simulink model "Restore_changes"  (R2022b)
settings: Solver=VariableStepAuto  StartTime=0.0  StopTime=10.0  RelTol=1e-3
undefined symbols (not defined in the file): Amplifier, DiscIntNeverNeededParam, K_d_yawrate, K_dsteering, k_speed, k_stanley
libraries: CarMaker4SL x19, simulink x7
settings Model: Creator=Admin  LastModifiedBy=Admin

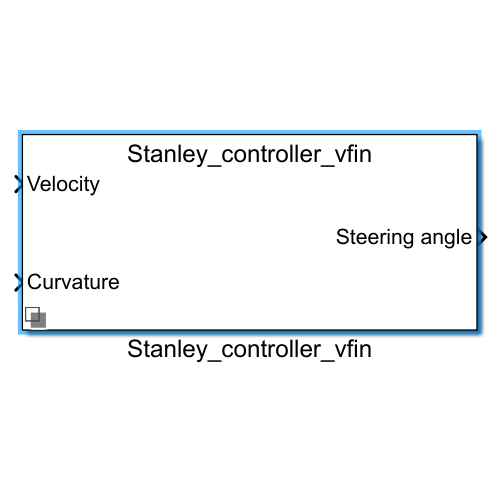
[thumbnail: Simulink's stored preview of the top-level diagram]
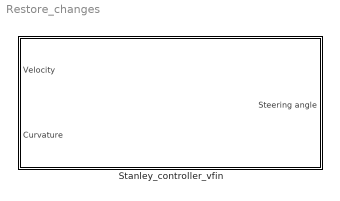
== system Restore_changes ==
  Stanley_controller_vfin : Subsystem  Variant=on  VariantControlMode=label  VariantControl=Choice  LabelModeActiveChoice=Choice

== system Restore_changes/Stanley_controller_vfin ==
  Velocity : Inport
  Curvature : Inport  Port=2
  Stanley_controller_vfin : Subsystem  Variant=on  VariantControlMode=label  VariantControl=Choice  LabelModeActiveChoice=Choice
  Steering angle : Outport

== system Restore_changes/Stanley_controller_vfin/Stanley_controller_vfin ==
  Velocity : Inport
  Curvature : Inport  Port=2
  Stanley_standfort controller : Subsystem  VariantControl=Choice
  Steering angle : Outport

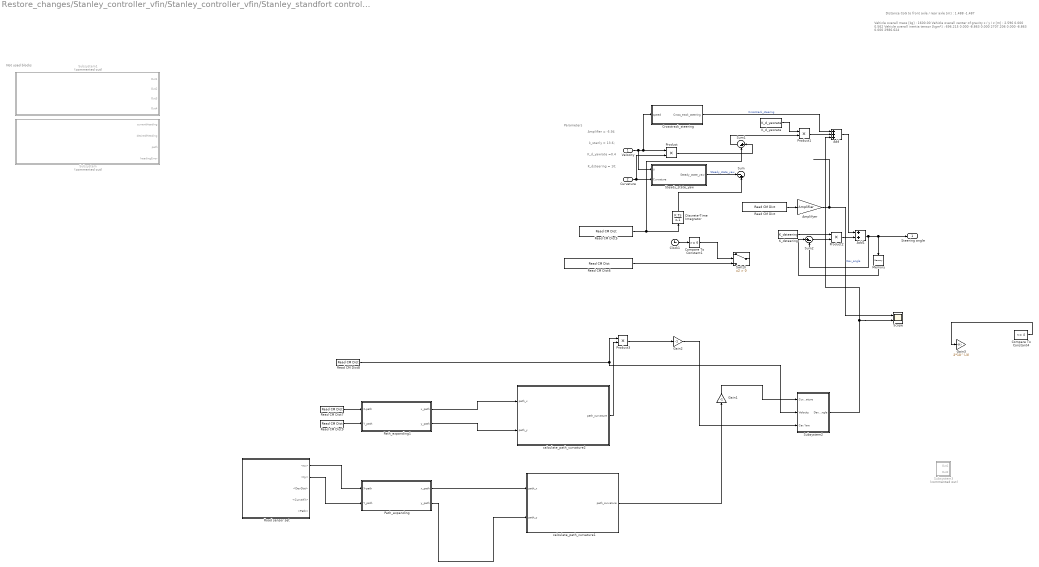
== system Restore_changes/Stanley_controller_vfin/Stanley_controller_vfin/Stanley_standfort controller ==
  note: Parameters
  note: K_dsteering = 10;
  note: Amplifier = -5.94
  note: K_d_yawrate =0.4
  note: Vehicle overall mass [kg] 	: 	1600.00
      |
      |  Vehicle overall center of gravity x / y / z [m] 	: 	2.596	0.000	0.562
      |
      |  Vehicle overall inertia tensor [kgm²] 	: 	696.215	0.000	-8.863
      |  	 									0.000	2707.206	0.000
      |  	 									-8.863	0.000	2986.624
  note: Distance CoG to front axle / rear axle [m] : 1.488 -1.487
  note: k_stanly = 13.6;
  note: Not used blocks
  Velocity : Inport
  Curvature : Inport  Port=2
  " Path_expanding" : Subsystem
  " Path_expanding1" : Subsystem
  Add : Sum  Inputs=+++
  Add1 : Sum
  Amplifyer : Gain  Gain=Amplifier
  Clock1 : Clock
  Compare To Constant1 : simulink/Logic and Bit Operations/Compare To Constant  relop=>=  const=6  OutDataTypeStr=boolean
  Compare To Constant4 : simulink/Logic and Bit Operations/Compare To Constant  relop=<=  const=4  OutDataTypeStr=boolean
  Crosstrack_steering : Subsystem
  Discrete-Time Integrator : DiscreteIntegrator  SampleTime=-1  ICPrevOutput=DiscIntNeverNeededParam  ICPrevScaledInput=DiscIntNeverNeededParam
  Gain1 : Gain  Gain=-1
  Gain2 : Gain  Gain=-1
  Gain3 : Gain  Gain=2*10^(-3)
  K_d_yawrate : Constant  Value=K_d_yawrate
  K_dsteering : Constant  Value=K_dsteering
  Memory : Memory  LinearizeAsDelay=on
  Product{,1..3} (4 alike) : Product
  Read CM Dict : CarMaker4SL/Read CM Dict  xname=Sensor.Road.VehSensor_0.Path.DevAng  xsync=off  xstime=Continuous
  Read CM Dict5 : CarMaker4SL/Read CM Dict  xname=Car.YawRate  xsync=off  xstime=Continuous
  Read CM Dict6 : CarMaker4SL/Read CM Dict  xname=Sensor.Road.VehSensor_0.Path.CurveXY  xsync=off  xstime=Continuous
  Read CM Dict7 : CarMaker4SL/Read CM Dict  xname=Car.Gen.tx  xsync=off  xstime=Continuous
  Read CM Dict8 : CarMaker4SL/Read CM Dict  xname=Vhcl.v  xsync=off  xstime=Continuous
  Read CM Dict9 : CarMaker4SL/Read CM Dict  xname=Car.Gen.ty  xsync=off  xstime=Continuous
  Road sensor set : Subsystem  Variant=on  VariantControlMode=label  VariantControl=Choice  LabelModeActiveChoice=Choice
  Scope : Scope  NumInputPorts=2
  Steady_state_yaw : Subsystem
  Subsystem : Subsystem  Commented=on
  Subsystem1 : Subsystem  Commented=on
  Subsystem2 : Subsystem
  Subsystem3 : Subsystem  Commented=on
  Sum : Sum  Inputs=|-+
  Sum1 : Sum  Inputs=|+-
  Sum2 : Sum  Inputs=|+-
  Switch : Switch  Criteria=u2 > Threshold  SaturateOnIntegerOverflow=off  InputSameDT=off
  calculate_path_curvature1 : MATLAB Function  TreatAsAtomicUnit=on  VariantControl=Choice
  calculate_path_curvature2 : MATLAB Function  TreatAsAtomicUnit=on  VariantControl=Choice
  Steering angle : Outport
  wires:
  Read CM Dict5/1 -> Discrete-Time Integrator/1, Sum1/2
  Velocity/1 -> Crosstrack_steering/1(speed), Product/1, Steady_state_yaw/1(V)
  Curvature/1 -> Steady_state_yaw/2(Curvature), Product/2
  Crosstrack_steering/1(Cross_track_steering) -> Add/1  "Crosstrack_steering"
  Product/1 -> Sum1/1
  Steady_state_yaw/1(Steady_state_yaw) -> Sum/1  "Steady_state_yaw"
  Discrete-Time Integrator/1 -> Sum/2
  Sum1/1 -> Product1/2
  K_d_yawrate/1 -> Product1/1
  Product1/1 -> Add/2
  Read CM Dict/1 -> Amplifyer/1
  Amplifyer/1 -> Scope/1  "Dev_angle"
  K_dsteering/1 -> Product2/1
  Sum2/1 -> Product2/2
  Add/1 -> Add1/1
  Product2/1 -> Add1/2
  Add1/1 -> Memory/1, Steering angle/1, Sum2/2
  Memory/1 -> Sum2/1
  Read CM Dict6/1 -> Switch/3
  Read CM Dict8/1 -> Product3/1, Subsystem2/2(Velocity)
  Road sensor set/1(<tx>) -> " Path_expanding"/1(X-path)
  Road sensor set/2(<ty>) -> " Path_expanding"/2(Y_path)
  " Path_expanding"/1(x_path) -> calculate_path_curvature1/1(path_x)
  " Path_expanding"/2(y_path) -> calculate_path_curvature1/2(path_y)
  calculate_path_curvature1/1(path_curvature) -> Gain1/1
  Subsystem2/1(Dev_angle) -> Add/3, Scope/2
  Clock1/1 -> Compare To Constant1/1
  Compare To Constant1/1 -> Switch/2
  Compare To Constant4/1 -> Gain3/1
  Gain1/1 -> Subsystem2/1(Curvature)
  " Path_expanding1"/1(x_path) -> calculate_path_curvature2/1(path_x)
  " Path_expanding1"/2(y_path) -> calculate_path_curvature2/2(path_y)
  Read CM Dict7/1 -> " Path_expanding1"/1(X-path)
  Read CM Dict9/1 -> " Path_expanding1"/2(Y_path)
  calculate_path_curvature2/1(path_curvature) -> Product3/2
  Product3/1 -> Gain2/1
  Gain2/1 -> Subsystem2/3(Car.Yaw)

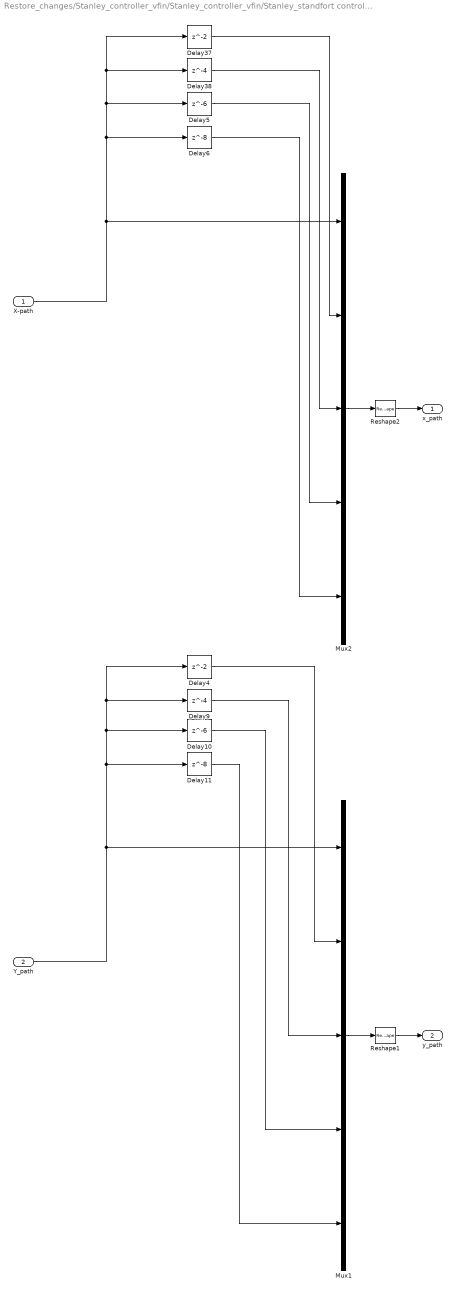
== system Restore_changes/Stanley_controller_vfin/Stanley_controller_vfin/Stanley_standfort controller/ Path_expanding ==
  X-path : Inport
  Y_path : Inport  Port=2
  Delay10 : Delay  DelayLength=6
  Delay11 : Delay  DelayLength=8
  Delay37 : Delay
  Delay38 : Delay  DelayLength=4
  Delay4 : Delay
  Delay5 : Delay  DelayLength=6
  Delay6 : Delay  DelayLength=8
  Delay9 : Delay  DelayLength=4
  Mux1 : Mux  Inputs=5
  Mux2 : Mux  Inputs=5
  Reshape1 : Reshape  OutputDimensionality=Customize  OutputDimensions=[1,5]
  Reshape2 : Reshape  OutputDimensionality=Customize  OutputDimensions=[1,5]
  x_path : Outport
  y_path : Outport  Port=2
  wires:
  X-path/1 -> Mux2/1, Delay38/1, Delay37/1, Delay5/1, Delay6/1
  Y_path/1 -> Mux1/1, Delay4/1, Delay9/1, Delay10/1, Delay11/1
  Delay5/1 -> Mux2/4
  Delay37/1 -> Mux2/2
  Delay6/1 -> Mux2/5
  Delay38/1 -> Mux2/3
  Mux1/1 -> Reshape1/1
  Reshape1/1 -> y_path/1
  Delay4/1 -> Mux1/2
  Delay9/1 -> Mux1/3
  Delay10/1 -> Mux1/4
  Delay11/1 -> Mux1/5
  Reshape2/1 -> x_path/1
  Mux2/1 -> Reshape2/1

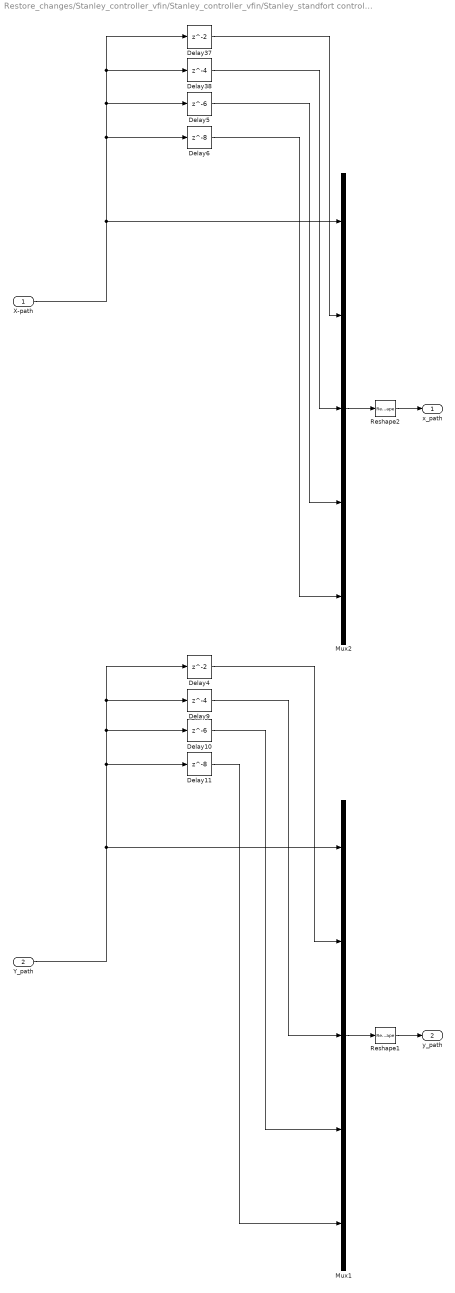
== system Restore_changes/Stanley_controller_vfin/Stanley_controller_vfin/Stanley_standfort controller/ Path_expanding1 ==
  X-path : Inport
  Y_path : Inport  Port=2
  Delay10 : Delay  DelayLength=6
  Delay11 : Delay  DelayLength=8
  Delay37 : Delay
  Delay38 : Delay  DelayLength=4
  Delay4 : Delay
  Delay5 : Delay  DelayLength=6
  Delay6 : Delay  DelayLength=8
  Delay9 : Delay  DelayLength=4
  Mux1 : Mux  Inputs=5
  Mux2 : Mux  Inputs=5
  Reshape1 : Reshape  OutputDimensionality=Customize  OutputDimensions=[1,5]
  Reshape2 : Reshape  OutputDimensionality=Customize  OutputDimensions=[1,5]
  x_path : Outport
  y_path : Outport  Port=2
  wires:
  Mux2/1 -> Reshape2/1
  Reshape2/1 -> x_path/1
  Delay11/1 -> Mux1/5
  Delay10/1 -> Mux1/4
  Delay9/1 -> Mux1/3
  Delay4/1 -> Mux1/2
  Reshape1/1 -> y_path/1
  Mux1/1 -> Reshape1/1
  Delay38/1 -> Mux2/3
  Delay6/1 -> Mux2/5
  Delay37/1 -> Mux2/2
  Delay5/1 -> Mux2/4
  Y_path/1 -> Delay11/1, Delay10/1, Delay9/1, Delay4/1, Mux1/1
  X-path/1 -> Delay6/1, Delay5/1, Delay37/1, Delay38/1, Mux2/1

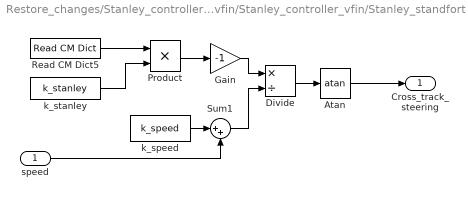
== system Restore_changes/Stanley_controller_vfin/Stanley_controller_vfin/Stanley_standfort controller/Crosstrack_steering ==
  speed : Inport
  Atan : Trigonometry  Operator=atan
  Divide : Product  Inputs=*/
  Gain : Gain  Gain=-1
  Product : Product
  Read CM Dict5 : CarMaker4SL/Read CM Dict  xname=Car.Road.Path.DevDist  xsync=off  xstime=Continuous
  Sum1 : Sum  Inputs=|++
  k_speed : Constant  Value=k_speed
  k_stanley : Constant  Value=k_stanley
  Cross_track_steering : Outport
  wires:
  Atan/1 -> Cross_track_steering/1
  Divide/1 -> Atan/1
  k_speed/1 -> Sum1/1
  speed/1 -> Sum1/2
  k_stanley/1 -> Product/2
  Sum1/1 -> Divide/2
  Product/1 -> Gain/1
  Read CM Dict5/1 -> Product/1
  Gain/1 -> Divide/1

== system Restore_changes/Stanley_controller_vfin/Stanley_controller_vfin/Stanley_standfort controller/Road sensor set ==
  Road sensor set : Subsystem  VariantControl=Choice
  <tx> : Outport
  <ty> : Outport  Port=2
  <DevDist> : Outport  Port=3
  <CurveXY> : Outport  Port=4
  <Path> : Outport  Port=5

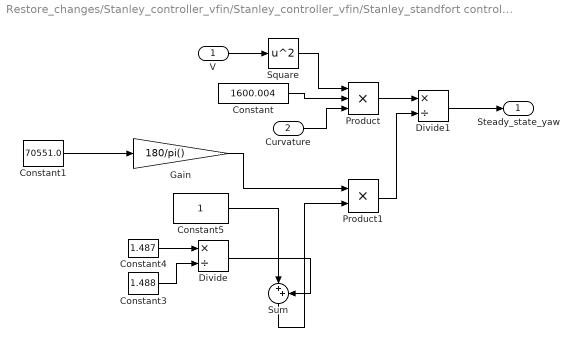
== system Restore_changes/Stanley_controller_vfin/Stanley_controller_vfin/Stanley_standfort controller/Steady_state_yaw ==
  V : Inport
  Curvature : Inport  Port=2
  Constant : Constant  Value=1600.004
  Constant1 : Constant  Value=70551.0
  Constant3 : Constant  Value=1.488
  Constant4 : Constant  Value=1.487
  Constant5 : Constant
  Divide : Product  Inputs=*/
  Divide1 : Product  Inputs=*/
  Gain : Gain  Gain=180/pi()
  Product : Product  Inputs=3
  Product1 : Product
  Square : Math  Operator=square
  Sum : Sum  Inputs=|++
  Steady_state_yaw : Outport
  wires:
  Square/1 -> Product/1
  Constant4/1 -> Divide/1
  Constant5/1 -> Sum/1
  Constant3/1 -> Divide/2
  V/1 -> Square/1
  Divide/1 -> Sum/2
  Sum/1 -> Product1/2
  Constant/1 -> Product/2
  Curvature/1 -> Product/3
  Constant1/1 -> Gain/1
  Product/1 -> Divide1/1
  Product1/1 -> Divide1/2
  Divide1/1 -> Steady_state_yaw/1
  Gain/1 -> Product1/1

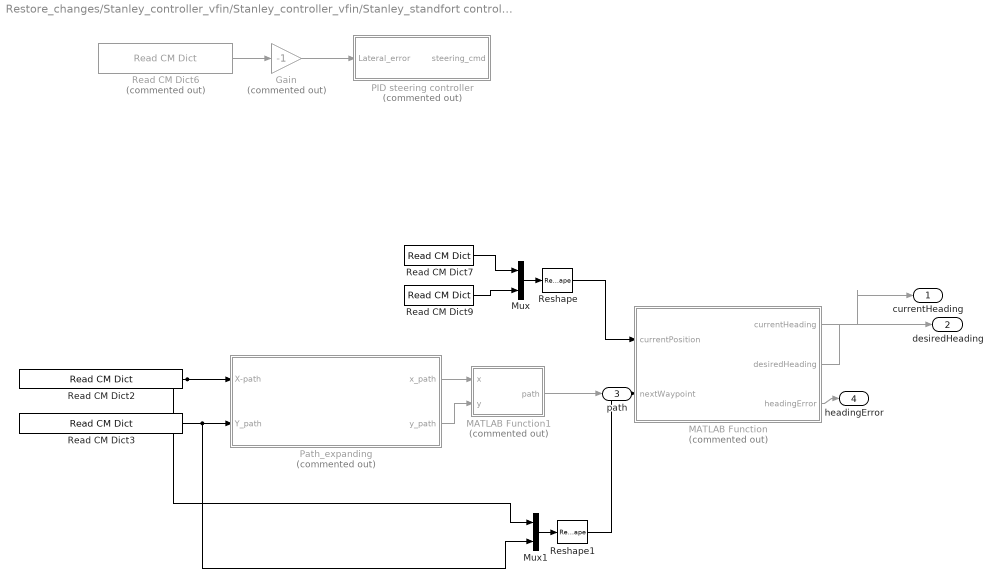
== system Restore_changes/Stanley_controller_vfin/Stanley_controller_vfin/Stanley_standfort controller/Subsystem ==
  " Path_expanding" : Subsystem  Commented=on
  Gain : Gain  Commented=on  Gain=-1
  MATLAB Function : MATLAB Function  Commented=on  TreatAsAtomicUnit=on
  MATLAB Function1 : MATLAB Function  Commented=on  TreatAsAtomicUnit=on
  Mux : Mux  Inputs=2
  Mux1 : Mux  Inputs=2
  PID steering controller : Subsystem  Commented=on
  Read CM Dict2 : CarMaker4SL/Read CM Dict  xname=Sensor.Road.VehSensor_0.Path.tx  xsync=off  xstime=Continuous
  Read CM Dict3 : CarMaker4SL/Read CM Dict  xname=Sensor.Road.VehSensor_0.Path.ty  xsync=off  xstime=Continuous
  Read CM Dict6 : CarMaker4SL/Read CM Dict  Commented=on  xname=Car.Road.Path.DevDist  xsync=off  xstime=Continuous
  Read CM Dict7 : CarMaker4SL/Read CM Dict  xname=Car.Road.tx  xsync=off  xstime=Continuous
  Read CM Dict9 : CarMaker4SL/Read CM Dict  xname=Car.Gen.ty  xsync=off  xstime=Continuous
  Reshape : Reshape  OutputDimensionality=Customize  OutputDimensions=[1,2]
  Reshape1 : Reshape  OutputDimensionality=Customize  OutputDimensions=[1,2]
  currentHeading : Outport
  desiredHeading : Outport  Port=2
  path : Outport  Port=3
  headingError : Outport  Port=4
  wires:
  Read CM Dict2/1 -> Mux1/1, " Path_expanding"/1(X-path)
  Reshape/1 -> MATLAB Function/1(currentPosition)
  MATLAB Function/1(currentHeading) -> currentHeading/1
  Mux1/1 -> Reshape1/1
  Read CM Dict3/1 -> Mux1/2, " Path_expanding"/2(Y_path)
  Mux/1 -> Reshape/1
  MATLAB Function1/1(path) -> path/1
  " Path_expanding"/2(y_path) -> MATLAB Function1/2(y)
  " Path_expanding"/1(x_path) -> MATLAB Function1/1(x)
  Read CM Dict9/1 -> Mux/2
  MATLAB Function/2(desiredHeading) -> desiredHeading/1
  Reshape1/1 -> MATLAB Function/2(nextWaypoint)
  Read CM Dict7/1 -> Mux/1
  MATLAB Function/3(headingError) -> headingError/1
  Read CM Dict6/1 -> Gain/1
  Gain/1 -> PID steering controller/1(Lateral_error)

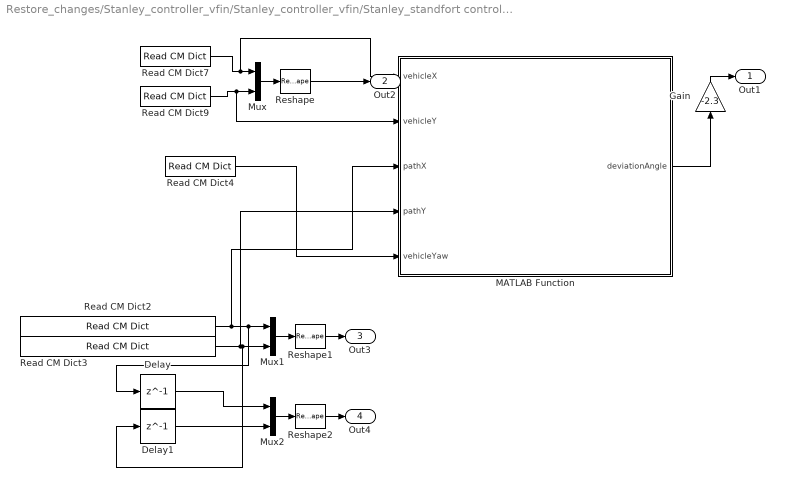
== system Restore_changes/Stanley_controller_vfin/Stanley_controller_vfin/Stanley_standfort controller/Subsystem1 ==
  Delay : Delay  DelayLength=1
  Delay1 : Delay  DelayLength=1
  Gain : Gain  Gain=-2.3
  MATLAB Function : MATLAB Function  TreatAsAtomicUnit=on
  Mux : Mux  Inputs=2
  Mux1 : Mux  Inputs=2
  Mux2 : Mux  Inputs=2
  Read CM Dict2 : CarMaker4SL/Read CM Dict  xname=Sensor.Road.VehSensor_0.Path.tx  xsync=off  xstime=Continuous
  Read CM Dict3 : CarMaker4SL/Read CM Dict  xname=Sensor.Road.VehSensor_0.Path.ty  xsync=off  xstime=Continuous
  Read CM Dict4 : CarMaker4SL/Read CM Dict  xname=Car.Yaw  xsync=off  xstime=Continuous
  Read CM Dict7 : CarMaker4SL/Read CM Dict  xname=Car.Gen.tx  xsync=off  xstime=Continuous
  Read CM Dict9 : CarMaker4SL/Read CM Dict  xname=Car.Gen.ty  xsync=off  xstime=Continuous
  Reshape : Reshape  OutputDimensionality=Customize  OutputDimensions=[1,2]
  Reshape1 : Reshape  OutputDimensionality=Customize  OutputDimensions=[1,2]
  Reshape2 : Reshape  OutputDimensionality=Customize  OutputDimensions=[1,2]
  Out1 : Outport
  Out2 : Outport  Port=2
  Out3 : Outport  Port=3
  Out4 : Outport  Port=4
  wires:
  Read CM Dict7/1 -> MATLAB Function/1(vehicleX), Mux/1
  Read CM Dict2/1 -> MATLAB Function/3(pathX), Delay/1, Mux1/1
  Mux1/1 -> Reshape1/1
  Read CM Dict9/1 -> MATLAB Function/2(vehicleY), Mux/2
  MATLAB Function/1(deviationAngle) -> Gain/1
  Read CM Dict3/1 -> MATLAB Function/4(pathY), Delay1/1, Mux1/2
  Mux/1 -> Reshape/1
  Read CM Dict4/1 -> MATLAB Function/5(vehicleYaw)
  Mux2/1 -> Reshape2/1
  Reshape2/1 -> Out4/1
  Reshape/1 -> Out2/1
  Delay/1 -> Mux2/1
  Delay1/1 -> Mux2/2
  Gain/1 -> Out1/1
  Reshape1/1 -> Out3/1

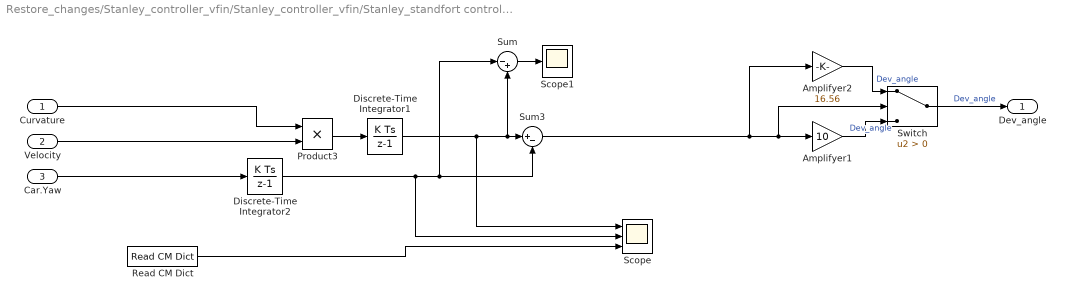
== system Restore_changes/Stanley_controller_vfin/Stanley_controller_vfin/Stanley_standfort controller/Subsystem2 ==
  Curvature : Inport
  Velocity : Inport  Port=2
  Car.Yaw : Inport  Port=3
  Amplifyer1 : Gain  Gain=10
  Amplifyer2 : Gain  Gain=16.56
  Discrete-Time Integrator1 : DiscreteIntegrator  SampleTime=-1  ICPrevOutput=DiscIntNeverNeededParam  ICPrevScaledInput=DiscIntNeverNeededParam
  Discrete-Time Integrator2 : DiscreteIntegrator  SampleTime=-1  ICPrevOutput=DiscIntNeverNeededParam  ICPrevScaledInput=DiscIntNeverNeededParam
  Product3 : Product
  Read CM Dict : CarMaker4SL/Read CM Dict  xname=Car.Yaw  xsync=off  xstime=Continuous
  Scope : Scope  NumInputPorts=3
  Scope1 : Scope
  Sum : Sum  Inputs=|-+
  Sum3 : Sum  Inputs=|+-
  Switch : Switch  Criteria=u2 > Threshold  SaturateOnIntegerOverflow=off  InputSameDT=off
  Dev_angle : Outport
  wires:
  Sum3/1 -> Amplifyer1/1, Switch/2, Amplifyer2/1
  Amplifyer2/1 -> Switch/1  "Dev_angle"
  Switch/1 -> Dev_angle/1  "Dev_angle"
  Product3/1 -> Discrete-Time Integrator1/1
  Amplifyer1/1 -> Switch/3  "Dev_angle"
  Car.Yaw/1 -> Discrete-Time Integrator2/1
  Curvature/1 -> Product3/1
  Velocity/1 -> Product3/2
  Discrete-Time Integrator1/1 -> Sum/2, Sum3/1, Scope/1
  Discrete-Time Integrator2/1 -> Sum/1, Sum3/2, Scope/2
  Read CM Dict/1 -> Scope/3
  Sum/1 -> Scope1/1

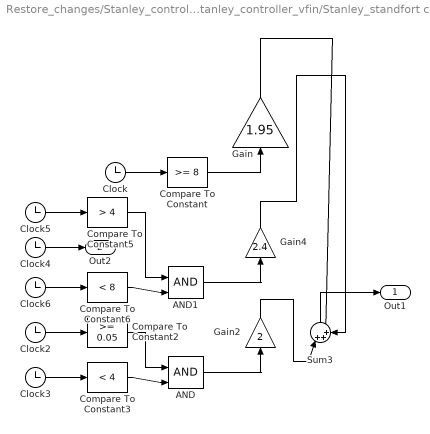
== system Restore_changes/Stanley_controller_vfin/Stanley_controller_vfin/Stanley_standfort controller/Subsystem3 ==
  AND : Logic  IconShape=distinctive  AllPortsSameDT=off  OutDataTypeStr=boolean
  AND1 : Logic  IconShape=distinctive  AllPortsSameDT=off  OutDataTypeStr=boolean
  Clock{,2..6} (6 alike) : Clock
  Compare To Constant : simulink/Logic and Bit Operations/Compare To Constant  relop=>=  const=8  OutDataTypeStr=boolean
  Compare To Constant2 : simulink/Logic and Bit Operations/Compare To Constant  relop=>=  const=0.05  OutDataTypeStr=boolean
  Compare To Constant3 : simulink/Logic and Bit Operations/Compare To Constant  relop=<  const=4  OutDataTypeStr=boolean
  Compare To Constant5 : simulink/Logic and Bit Operations/Compare To Constant  relop=>  const=4  OutDataTypeStr=boolean
  Compare To Constant6 : simulink/Logic and Bit Operations/Compare To Constant  relop=<  const=8  OutDataTypeStr=boolean
  Gain : Gain  Gain=1.95
  Gain2 : Gain  Gain=2
  Gain4 : Gain  Gain=2.4
  Sum3 : Sum  Inputs=|+++
  Out1 : Outport
  Out2 : Outport  Port=2
  wires:
  Clock4/1 -> Out2/1
  Clock5/1 -> Compare To Constant5/1
  Clock6/1 -> Compare To Constant6/1
  Compare To Constant6/1 -> AND1/2
  Clock2/1 -> Compare To Constant2/1
  Clock3/1 -> Compare To Constant3/1
  Clock/1 -> Compare To Constant/1
  Compare To Constant5/1 -> AND1/1
  AND1/1 -> Gain4/1
  Compare To Constant2/1 -> AND/1
  Compare To Constant3/1 -> AND/2
  Compare To Constant/1 -> Gain/1
  AND/1 -> Gain2/1
  Gain/1 -> Sum3/2
  Gain4/1 -> Sum3/3
  Gain2/1 -> Sum3/1
  Sum3/1 -> Out1/1

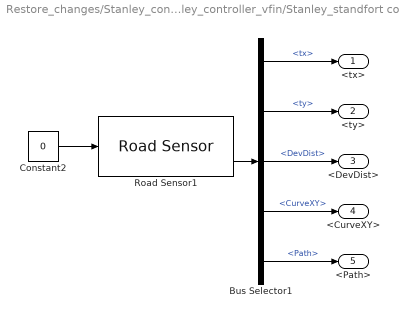
== system Restore_changes/Stanley_controller_vfin/Stanley_controller_vfin/Stanley_standfort controller/Road sensor set/Road sensor set ==
  Bus Selector1 : BusSelector  OutputSignals=Path.tx,Path.ty,Path.DevDist,Path.CurveXY,Path
  Constant2 : Constant  Value=0
  Road Sensor1 : CarMaker4SL/Sensors/Road Sensor  xname=0  xstime=Continuous
      settings: SourceProductName=CarMaker4SL
  <tx> : Outport
  <ty> : Outport  Port=2
  <DevDist> : Outport  Port=3
  <CurveXY> : Outport  Port=4
  <Path> : Outport  Port=5
  wires:
  Constant2/1 -> Road Sensor1/1
  Road Sensor1/2 -> Bus Selector1/1
  Bus Selector1/5 -> <Path>/1  "<Path>"
  Bus Selector1/1 -> <tx>/1  "<tx>"
  Bus Selector1/4 -> <CurveXY>/1  "<CurveXY>"
  Bus Selector1/2 -> <ty>/1  "<ty>"
  Bus Selector1/3 -> <DevDist>/1  "<DevDist>"

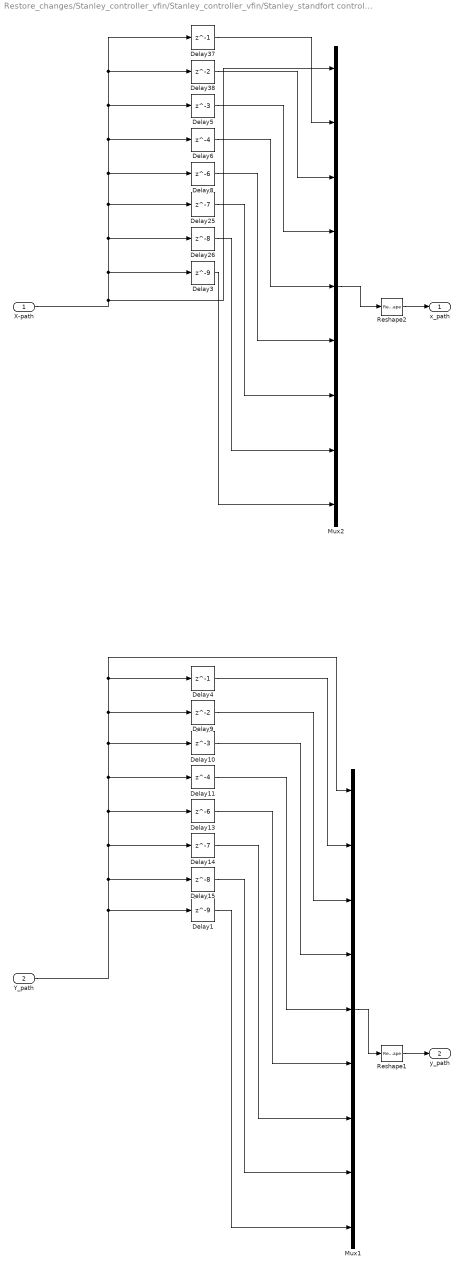
== system Restore_changes/Stanley_controller_vfin/Stanley_controller_vfin/Stanley_standfort controller/Subsystem/ Path_expanding ==
  X-path : Inport
  Y_path : Inport  Port=2
  Delay1 : Delay  DelayLength=9
  Delay10 : Delay  DelayLength=3
  Delay11 : Delay  DelayLength=4
  Delay13 : Delay  DelayLength=6
  Delay14 : Delay  DelayLength=7
  Delay15 : Delay  DelayLength=8
  Delay25 : Delay  DelayLength=7
  Delay26 : Delay  DelayLength=8
  Delay3 : Delay  DelayLength=9
  Delay37 : Delay  DelayLength=1
  Delay38 : Delay
  Delay4 : Delay  DelayLength=1
  Delay5 : Delay  DelayLength=3
  Delay6 : Delay  DelayLength=4
  Delay8 : Delay  DelayLength=6
  Delay9 : Delay
  Mux1 : Mux  Inputs=9
  Mux2 : Mux  Inputs=9
  Reshape1 : Reshape  OutputDimensionality=Customize  OutputDimensions=[1,9]
  Reshape2 : Reshape  OutputDimensionality=Customize  OutputDimensions=[1,9]
  x_path : Outport
  y_path : Outport  Port=2
  wires:
  X-path/1 -> Mux2/1, Delay38/1, Delay37/1, Delay5/1, Delay6/1, Delay8/1, Delay25/1, Delay26/1, Delay3/1
  Delay25/1 -> Mux2/7
  Y_path/1 -> Mux1/1, Delay4/1, Delay9/1, Delay10/1, Delay11/1, Delay13/1, Delay14/1, Delay15/1, Delay1/1
  Delay5/1 -> Mux2/4
  Delay37/1 -> Mux2/2
  Delay6/1 -> Mux2/5
  Delay38/1 -> Mux2/3
  Delay8/1 -> Mux2/6
  Delay26/1 -> Mux2/8
  Mux1/1 -> Reshape1/1
  Delay1/1 -> Mux1/9
  Delay15/1 -> Mux1/8
  Reshape1/1 -> y_path/1
  Delay4/1 -> Mux1/2
  Delay9/1 -> Mux1/3
  Delay10/1 -> Mux1/4
  Delay11/1 -> Mux1/5
  Delay13/1 -> Mux1/6
  Reshape2/1 -> x_path/1
  Delay14/1 -> Mux1/7
  Mux2/1 -> Reshape2/1
  Delay3/1 -> Mux2/9

== system Restore_changes/Stanley_controller_vfin/Stanley_controller_vfin/Stanley_standfort controller/Subsystem/PID steering controller ==
  Lateral_error : Inport
  Add : Sum  Inputs=+++
  Derivative : Derivative
  Discrete-Time Integrator : DiscreteIntegrator  SampleTime=-1  ICPrevOutput=DiscIntNeverNeededParam  ICPrevScaledInput=DiscIntNeverNeededParam
  Gain : Gain  Gain=0.6
  Gain1 : Gain  Gain=0.9
  Gain2 : Gain  Gain=0.4
  steering_cmd : Outport
  wires:
  Lateral_error/1 -> Gain1/1, Gain/1, Gain2/1
  Discrete-Time Integrator/1 -> Add/1
  Gain2/1 -> Derivative/1
  Gain1/1 -> Discrete-Time Integrator/1
  Gain/1 -> Add/2
  Derivative/1 -> Add/3
  Add/1 -> steering_cmd/1

== matlab function Restore_changes/Stanley_controller_vfin/Stanley_controller_vfin/Stanley_standfort controller/Subsystem/MATLAB Function ==
  data: currentPosition input; currentHeading output; nextWaypoint input; desiredHeading output; headingError output
function [currentHeading, desiredHeading, headingError] = calculateHeadingError(currentPosition, nextWaypoint)
    % Calculate current heading, desired heading, and heading error for Stanley controller
    % Inputs:
    %   - currentPosition: Current position of the vehicle [x, y] (single points)
    %   - nextWaypoint: Next waypoint on the path [x, y]
    % Outputs:
    %   - currentHeading: Current heading of the vehicle (in radians)
    %   - desiredHeading: Desired heading or reference angle (in radians)
    %   - headingError: Heading error (in radians)
    function angle = wrapToPi(angle)
    % Wrap angle to the range [-pi, pi]
    angle = mod(angle + pi, 2 * pi) - pi;
    end
    % Extract x and y coordinates from the current position
    x = currentPosition(1);
    y = currentPosition(2);
    
    % Calculate the vector from the vehicle to the next waypoint
    headingVector = nextWaypoint - [x, y];

    % Calculate the current heading
    currentHeading = atan2(headingVector(2), headingVector(1));
    disp(currentHeading)
    disp('next')
    % Calculate the desired heading (heading of the vector between the current position and next waypoint)
    desiredHeading = atan2(nextWaypoint(2) - y, nextWaypoint(1) - x);
    disp(desiredHeading)
    % Calculate heading error
    headingError = wrapToPi(desiredHeading - currentHeading);
end

== matlab function Restore_changes/Stanley_controller_vfin/Stanley_controller_vfin/Stanley_standfort controller/Subsystem/MATLAB Function1 ==
  data: x input; path output; y input
function path = fcn(x , y)
path = [x;y];
end

== matlab function Restore_changes/Stanley_controller_vfin/Stanley_controller_vfin/Stanley_standfort controller/Subsystem1/MATLAB Function ==
  data: vehicleX input; deviationAngle output; vehicleY input; pathX input; pathY input; vehicleYaw input
function deviationAngle = calculateDeviationAngle(vehicleX, vehicleY, pathX, pathY, vehicleYaw)
    % Calculate the vector from the vehicle to the path point
    vectorToPath = [pathX - vehicleX, pathY - vehicleY];

    % Calculate the angle between the vehicle's heading and the vector to the path point
    angleToPath = atan2(vectorToPath(2), vectorToPath(1));

    % Calculate the deviation angle
    deviationAngle = vehicleYaw - angleToPath;

    % Ensure the result is within the range [-pi, pi]
    deviationAngle = mod(deviationAngle + pi, 2*pi) - pi;
end

== matlab function Restore_changes/Stanley_controller_vfin/Stanley_controller_vfin/Stanley_standfort controller/calculate_path_curvature2 ==
  data: path_x input; path_curvature output; path_y input
function path_curvature = calculate_path_curvature(path_x, path_y)
    x = path_x;
    y = path_y;
    
    % First and second derivatives
    dx = gradient(x);
    dy = gradient(y);
    
    ddx = gradient(dx);
    ddy = gradient(dy);
    
    % Path curvature with a small constant added to the denominator
    epsilon = 1e-6; % small constant to avoid division by zero
    curvature_denominator = (dx.^2 + dy.^2).^(3/2) + epsilon;
    path_curvature = max((dx .* ddy - dy .* ddx) ./ curvature_denominator);
    
    % Smooth the curvature using a moving average
    %window_size = 5; % adjust the window size as needed
    %path_curvature = smoothdata(path_curvature, 'movmean', window_size);
end

== matlab function Restore_changes/Stanley_controller_vfin/Stanley_controller_vfin/Stanley_standfort controller/calculate_path_curvature1 ==
  data: path_x input; path_curvature output; path_y input
function path_curvature = calculate_path_curvature(path_x, path_y)
    x = path_x;
    y = path_y;
    
    % First and second derivatives
    dx = gradient(x);
    dy = gradient(y);
    
    ddx = gradient(dx);
    ddy = gradient(dy);
    
    % Path curvature with a small constant added to the denominator
    epsilon = 1e-6; % small constant to avoid division by zero
    curvature_denominator = (dx.^2 + dy.^2).^(3/2) + epsilon;
    path_curvature = max((dx .* ddy - dy .* ddx) ./ curvature_denominator);
    
    % Smooth the curvature using a moving average
    %window_size = 5; % adjust the window size as needed
    %path_curvature = smoothdata(path_curvature, 'movmean', window_size);
end
